simulink model "PS_Lab_Experiment4"  (R2015a)
settings: Solver=ode45  StartTime=0.0  StopTime=25  RelTol=1e-3
settings Model: Creator=student  LastModifiedBy=student

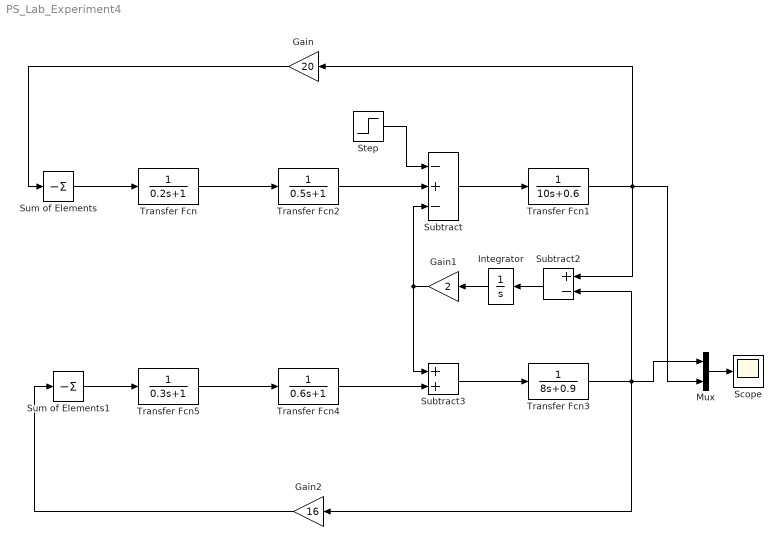
== system PS_Lab_Experiment4 ==
  Gain : Gain  Gain=20
  Gain1 : Gain  Gain=2
  Gain2 : Gain  Gain=16
  Integrator : Integrator
  Mux : Mux  Inputs=2
  Scope : Scope
  Step : Step  SampleTime=0
  Subtract : Sum  Inputs=-+-
  Subtract2 : Sum  Inputs=+-
  Subtract3 : Sum
  Sum of Elements : Sum  Inputs=-
  Sum of Elements1 : Sum  Inputs=-
  Transfer Fcn : TransferFcn  Denominator=[0.2 1]
  Transfer Fcn1 : TransferFcn  Denominator=[10 0.6]
  Transfer Fcn2 : TransferFcn  Denominator=[0.5 1]
  Transfer Fcn3 : TransferFcn  Denominator=[8 0.9]
  Transfer Fcn4 : TransferFcn  Denominator=[0.6 1]
  Transfer Fcn5 : TransferFcn  Denominator=[0.3 1]
  wires:
  Transfer Fcn2/1 -> Subtract/2
  Sum of Elements/1 -> Transfer Fcn/1
  Transfer Fcn/1 -> Transfer Fcn2/1
  Subtract/1 -> Transfer Fcn1/1
  Transfer Fcn1/1 -> Subtract2/1, Mux/2, Gain/1
  Step/1 -> Subtract/1
  Transfer Fcn3/1 -> Gain2/1, Mux/1, Subtract2/2
  Subtract3/1 -> Transfer Fcn3/1
  Subtract2/1 -> Integrator/1
  Gain1/1 -> Subtract3/1, Subtract/3
  Integrator/1 -> Gain1/1
  Transfer Fcn4/1 -> Subtract3/2
  Transfer Fcn5/1 -> Transfer Fcn4/1
  Gain/1 -> Sum of Elements/1
  Sum of Elements1/1 -> Transfer Fcn5/1
  Gain2/1 -> Sum of Elements1/1
  Mux/1 -> Scope/1
